simulink model "Analog_DSSS"  (R2017a)
settings: Solver=VariableStepAuto  StartTime=0.0  StopTime=100.0  RelTol=1e-3
libraries: dsparch4 x1, commseqgen3 x1, commutil2 x1
settings Model: Creator=rooki  LastModifiedBy=rooki

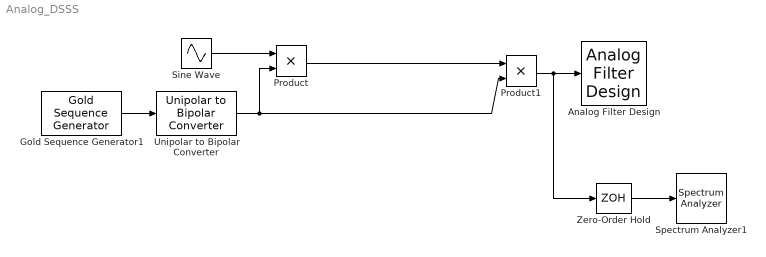
== system Analog_DSSS ==
  Analog Filter Design : dsparch4/Analog Filter Design  method=Butterworth  filttype=Lowpass  N=8  Wlo=10  Whi=80  Rp=2  Rs=40
  Gold Sequence Generator1 : commseqgen3/Gold Sequence Generator  genPoly1='z^6 + z + 1'  iniState1=[1 0 0 1 0 0]  genPoly2='z^6 + z^5 + z^2 + z + 1'  iniState2=[1 0 0 1 0 0]  index=0  shift=0  outVarSiz=off  maxOutSizeMode=Dialog parameter  maxOutSize=[10 1]  Ts=1/32  sampPerFrame=1  reset=off  outDataType=double
      settings: SourceProductName=Communications System Toolbox  SourceProductBaseCode=CM
  Product : Product
  Product1 : Product
  Sine Wave : Sin  SampleTime=0
  Spectrum Analyzer1 : SpectrumAnalyzer
  Unipolar to Bipolar Converter : commutil2/Unipolar to Bipolar Converter  M=2  polarity=Positive  dataType=Inherit via internal rule
      settings: SourceProductName=Communications System Toolbox
  Zero-Order Hold : ZeroOrderHold  SampleTime=-1
  wires:
  Sine Wave/1 -> Product/1
  Product/1 -> Product1/1
  Product1/1 -> Zero-Order Hold/1, Analog Filter Design/1
  Gold Sequence Generator1/1 -> Unipolar to Bipolar Converter/1
  Unipolar to Bipolar Converter/1 -> Product1/2, Product/2
  Zero-Order Hold/1 -> Spectrum Analyzer1/1
